simulink library "slc"  (Simulink 8.1)
settings: Solver=ode1  StartTime=0.0  StopTime=Inf  FixedStep=0.001  RelTol=1e-3
PostLoadFcn:
  | , if any(exist('dsrtsu_mdlpostloadfcn', 'file') == [2, 3, 6]), try dsrtsu_mdlpostloadfcn('Execute', bdroot); catch fprintf('Error in PostLoadFcn (dsrtsu_mdlpostloadfcn) for model "%s":\n %s\n', bdroot, lasterr); end, end,
libraries: ars x1, bts x1, dcl x1, tvb x1, tco x1
settings Model: DSRTSU_INTERNAL_RTI_VER=450  DSRTSU_INTERNAL_RTI_TYPE=rti1401  RTICANMMDATA=struct('GeneralSetupData',struct('modelroot','D:\ELN150201_TAIWAN\trunk\AdasDragon\software\sw_development\arch\app\acc','generalsettings',struct('filesettings',struct('destfolder',struct('Name','RTICANMM_FILES','Check',1),'buildfolder',struct('Name','.','Check',1),'AbsDestfolder',struct('Name','D:\ELN150201_TAIWAN\trunk\AdasDragon\software\sw_development\arch\app\acc\RTICANMM_FILES'),'AbsBuildfolder',struct('Name','D:\ELN150201_TAIWAN\trunk\AdasDragon\software\sw_development\arch\app\acc'))),'options',struct('addpaths',1,'rmpaths',1,'addtrcexclusion',logical(1),'cannavigator',struct('checkmonitoring',0),'show_usrtrc',0,'use_usrtrc',0),'advanced',struct('options',[1 1 1 1 1 1 1 1 1 1 1 1 1 1 1 1 1 1 1 1 1 1 1 1 1 1 1 1 1 1 1 1 1 1 1 1 1 1 1 1 1 1 1 1 1 1 1 1 1 1 1 1 1 1 1 1 1 1 1 1 1 1 1 1 1 1 1 1 1 1 1 1 1 1 1 1 1 1 1 1 1 1 1 1 1 1 1 1 1 1 1 1 1 1 1 1 1 1 1 1]),'MPSetup',{{}},'modelname','slc','block','slc'))  DSRTSU_INTERNAL_RTIFPGA=40  Creator=tescamilla  LastModifiedBy=AT015555

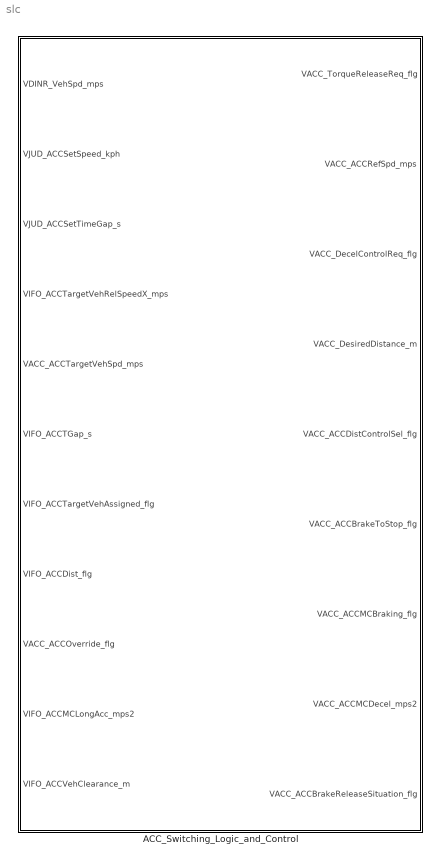
== system slc ==
  ACC_Switching_Logic_and_Control : Subsystem

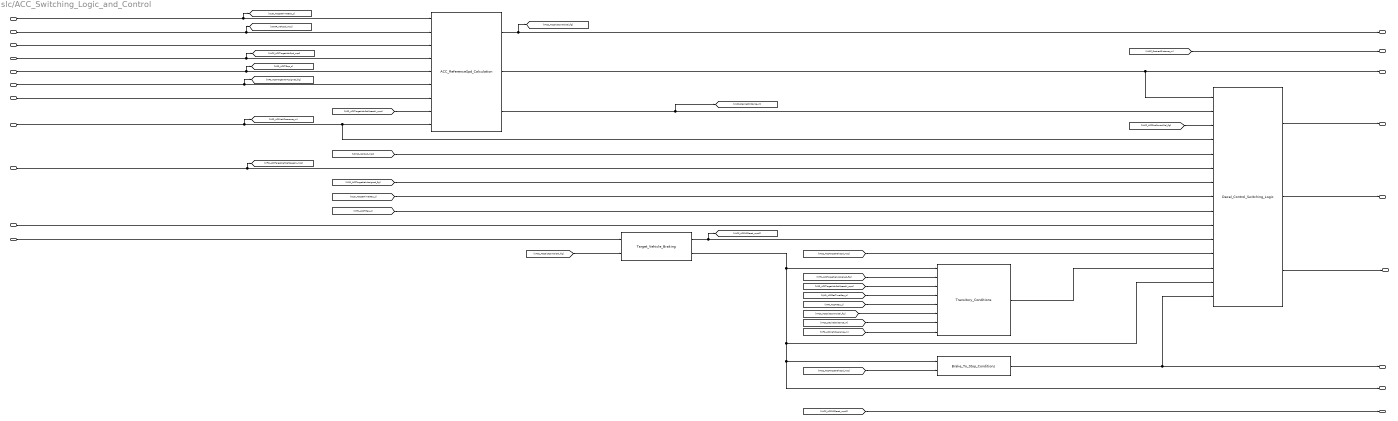
== system slc/ACC_Switching_Logic_and_Control ==
  VDINR_VehSpd_mps : Inport
  VJUD_ACCSetSpeed_kph : Inport  Port=2
  VJUD_ACCSetTimeGap_s : Inport  Port=3
  VIFO_ACCTargetVehRelSpeedX_mps : Inport  Port=4
  VACC_ACCTargetVehSpd_mps : Inport  Port=5
  VIFO_ACCTGap_s : Inport  Port=6
  VIFO_ACCTargetVehAssigned_flg : Inport  Port=7
  VIFO_ACCDist_flg : Inport  Port=8
  VACC_ACCOverride_flg : Inport  Port=9
  VIFO_ACCMCLongAcc_mps2 : Inport  Port=10
  VIFO_ACCVehClearance_m : Inport  Port=11
  ACC_ReferenceSpd_Calculation : ars/ACC_ReferenceSpd_Calculation
  Brake_To_Stop_Conditions : bts/Brake_To_Stop_Conditions
  Decel_Control_Switching_Logic : dcl/Decel_Control_Switching_Logic
  Target_Vehicle_Braking : tvb/Target_Vehicle_Braking
  Transitory_Conditions : tco/Transitory_Conditions
  VACC_TorqueReleaseReq_flg : Outport
  VACC_ACCRefSpd_mps : Outport  Port=2
  VACC_DecelControlReq_flg : Outport  Port=3
  VACC_DesiredDistance_m : Outport  Port=4
  VACC_ACCDistControlSel_flg : Outport  Port=5
  VACC_ACCBrakeToStop_flg : Outport  Port=6
  VACC_ACCMCBraking_flg : Outport  Port=7
  VACC_ACCMCDecel_mps2 : Outport  Port=8
  VACC_ACCBrakeReleaseSituation_flg : Outport  Port=9
  wires:
  Decel_Control_Switching_Logic/1 -> VACC_DecelControlReq_flg/1
  VIFO_ACCTargetVehRelSpeedX_mps/1 -> [VIFO_ACCTargetVehRelSpeedX_mps], Decel_Control_Switching_Logic/6
  VIFO_ACCTGap_s/1 -> ACC_ReferenceSpd_Calculation/5, [VIFO_ACCTGap_s]
  ACC_ReferenceSpd_Calculation/2 -> Decel_Control_Switching_Logic/1, VACC_ACCRefSpd_mps/1
  VJUD_ACCSetTimeGap_s/1 -> [VJUD_ACCSetTimeGap_s], ACC_ReferenceSpd_Calculation/1
  [VDINR_VehSpd_mps] -> Decel_Control_Switching_Logic/5
  VIFO_ACCVehClearance_m/1 -> [VIFO_ACCVehClearance_m], Decel_Control_Switching_Logic/4, ACC_ReferenceSpd_Calculation/9
  VACC_ACCTargetVehSpd_mps/1 -> ACC_ReferenceSpd_Calculation/4, [VACC_ACCTargetVehSpd_mps]
  VJUD_ACCSetSpeed_kph/1 -> ACC_ReferenceSpd_Calculation/3
  ACC_ReferenceSpd_Calculation/3 -> Decel_Control_Switching_Logic/2, [VACC_DesiredDistance_m]
  VDINR_VehSpd_mps/1 -> ACC_ReferenceSpd_Calculation/2, [VDINR_VehSpd_mps]
  VIFO_ACCTargetVehAssigned_flg/1 -> ACC_ReferenceSpd_Calculation/6, [VIFO_ACCTargetVehAssigned_flg]
  [VACC_DesiredDistance_m] -> VACC_DesiredDistance_m/1
  Decel_Control_Switching_Logic/2 -> VACC_TorqueReleaseReq_flg/1
  [VIFO_ACCTargetVehAssigned_flg] -> Transitory_Conditions/2
  [VIFO_ACCTGap_s] -> Decel_Control_Switching_Logic/9
  [VJUD_ACCSetTimeGap_s] -> Decel_Control_Switching_Logic/8
  [VIFO_ACCTargetVehAssigned_flg] -> Decel_Control_Switching_Logic/7
  VIFO_ACCDist_flg/1 -> ACC_ReferenceSpd_Calculation/7
  VACC_ACCOverride_flg/1 -> Decel_Control_Switching_Logic/10
  ACC_ReferenceSpd_Calculation/1 -> [VACC_ACCDistControlSel_flg], VACC_ACCDistControlSel_flg/1
  [VACC_ACCDistControlSel_flg] -> Decel_Control_Switching_Logic/3
  [VJUD_ACCSetTimeGap_s] -> Transitory_Conditions/4
  [VIFO_ACCTGap_s] -> Transitory_Conditions/5
  [VIFO_ACCTargetVehRelSpeedX_mps] -> Transitory_Conditions/3
  Transitory_Conditions/1 -> Decel_Control_Switching_Logic/13
  [VACC_DesiredDistance_m] -> Transitory_Conditions/7
  [VACC_ACCDistControlSel_flg] -> Transitory_Conditions/6
  [VIFO_ACCVehClearance_m] -> Transitory_Conditions/8
  [VIFO_ACCTargetVehRelSpeedX_mps] -> ACC_ReferenceSpd_Calculation/8
  [VACC_ACCTargetVehSpd_mps] -> Brake_To_Stop_Conditions/2
  Brake_To_Stop_Conditions/1 -> Decel_Control_Switching_Logic/15, VACC_ACCBrakeToStop_flg/1
  [VACC_ACCTargetVehSpd_mps] -> Decel_Control_Switching_Logic/12
  Target_Vehicle_Braking/1 -> [VACC_ACCMCDecel_mps2], Decel_Control_Switching_Logic/11
  Target_Vehicle_Braking/2 -> Decel_Control_Switching_Logic/14, VACC_ACCMCBraking_flg/1, Brake_To_Stop_Conditions/1, Transitory_Conditions/1
  VIFO_ACCMCLongAcc_mps2/1 -> Target_Vehicle_Braking/1
  [VACC_ACCDistControlSel_flg] -> Target_Vehicle_Braking/2
  [VACC_ACCMCDecel_mps2] -> VACC_ACCMCDecel_mps2/1
  Decel_Control_Switching_Logic/3 -> VACC_ACCBrakeReleaseSituation_flg/1
